simulink model "PowerAnalyserModel"  (R2026a)
settings: Solver=FixedStepAuto  StopTime=0.27  FixedStep=1e-5
libraries: eeRmsMeasurement x2, simulink x1
settings Model: Creator=Giulia  LastModifiedBy=Giulia

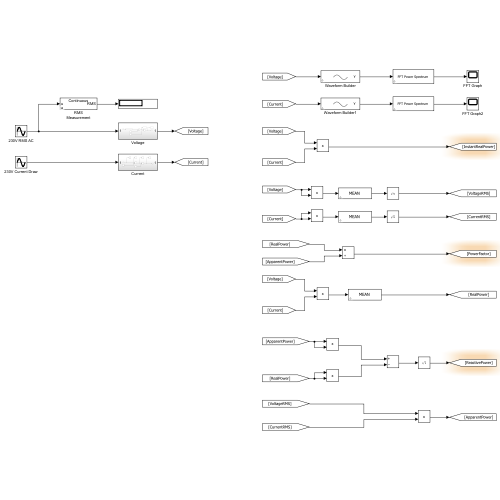
[thumbnail: Simulink's stored preview of the top-level diagram]
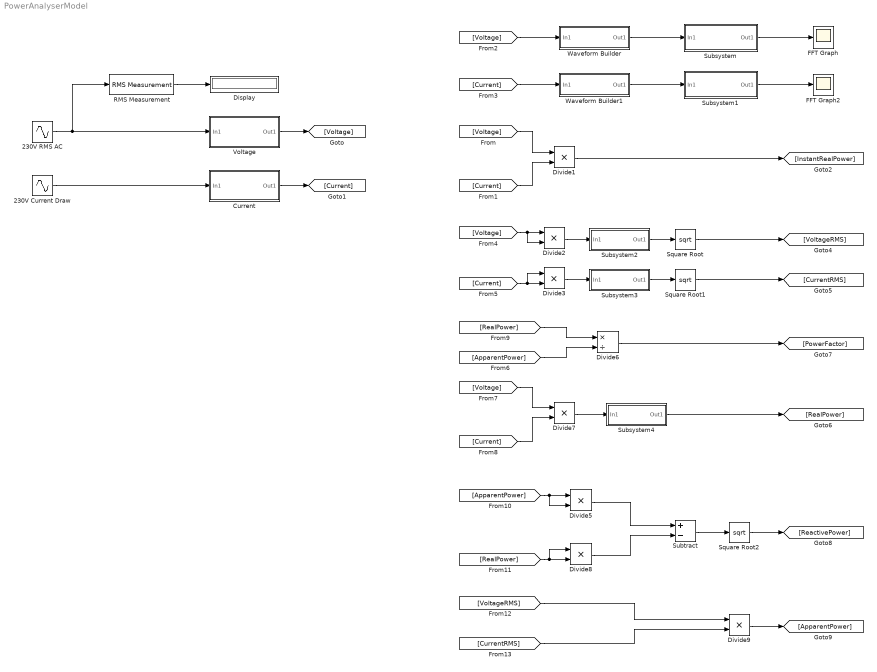
== system PowerAnalyserModel ==
  230V Current Draw : Sin  Amplitude=0.003  Frequency=50*pi*2  SampleTime=0
  230V RMS AC : Sin  Amplitude=325  Frequency=50*pi*2  SampleTime=0
  Current : Subsystem
  Display : Display
  Divide{1..3,5,7..9} (7 alike) : Product  Inputs=**
  Divide6 : Product  Inputs=*/
  FFT Graph : Scope
      settings: DataLoggingVariableName=ScopeData4
  FFT Graph2 : Scope
      settings: DataLoggingVariableName=ScopeData5
  RMS Measurement : eeRmsMeasurement/RMS Measurement  LabelModeActiveChoice=Total  F=50  SpecifyHarmonics=off  K=[0 1 2]  Ts=0
      settings: LibrarySourceBlock=|
      | ee_sl_lib/Measurements/RMS
      | Measurement
  Square Root : Sqrt
  Square Root1 : Sqrt
  Square Root2 : Sqrt
  Subsystem : Subsystem
  Subsystem1 : Subsystem
  Subsystem2 : Subsystem
  Subsystem3 : Subsystem
  Subsystem4 : Subsystem
  Subtract : Sum  Inputs=+-
  Voltage : Subsystem
  Waveform Builder : Subsystem
  Waveform Builder1 : Subsystem
  wires:
  230V RMS AC/1 -> Voltage/1(In1), RMS Measurement/1
  RMS Measurement/1 -> Display/1
  230V Current Draw/1 -> Current/1(In1)
  Voltage/1(Out1) -> [Voltage]
  Current/1(Out1) -> [Current]
  [Voltage] -> Divide1/1
  [Current] -> Divide1/2
  Divide1/1 -> [InstantRealPower]
  [Voltage] -> Waveform Builder/1(In1)
  Waveform Builder/1(Out1) -> Subsystem/1(In1)
  Subsystem/1(Out1) -> FFT Graph/1
  [Current] -> Waveform Builder1/1(In1)
  Waveform Builder1/1(Out1) -> Subsystem1/1(In1)
  Subsystem1/1(Out1) -> FFT Graph2/1
  [Voltage] -> Divide2/2, Divide2/1
  [Current] -> Divide3/1, Divide3/2
  Divide2/1 -> Subsystem2/1(In1)
  Divide3/1 -> Subsystem3/1(In1)
  Subsystem3/1(Out1) -> Square Root1/1
  Subsystem2/1(Out1) -> Square Root/1
  [ApparentPower] -> Divide6/2
  [Voltage] -> Divide7/1
  [Current] -> Divide7/2
  Divide7/1 -> Subsystem4/1(In1)
  Subsystem4/1(Out1) -> [RealPower]
  Square Root/1 -> [VoltageRMS]
  Square Root1/1 -> [CurrentRMS]
  [RealPower] -> Divide6/1
  Divide6/1 -> [PowerFactor]
  Square Root2/1 -> [ReactivePower]
  Subtract/1 -> Square Root2/1
  [ApparentPower] -> Divide5/2, Divide5/1
  Divide5/1 -> Subtract/1
  [RealPower] -> Divide8/1, Divide8/2
  Divide8/1 -> Subtract/2
  Divide9/1 -> [ApparentPower]
  [VoltageRMS] -> Divide9/1
  [CurrentRMS] -> Divide9/2

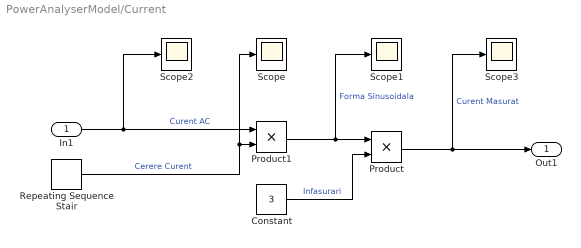
== system PowerAnalyserModel/Current ==
  In1 : Inport
  Constant : Constant  Value=3
  Product : Product
  Product1 : Product
  Repeating Sequence Stair : simulink/Sources/Repeating Sequence Stair  OutValues=[0 1 2 3 4 5 6 7 8 9 10 11 12 13].'  tsamp=0.02  OutMin=[]  OutMax=[]  OutDataTypeStr=double  OutputDataTypeScalingMode=double  OutDataType=fixdt(0,8)  ConRadixGroup=Best Precision: Vector-wise  OutScaling=2^-12
  Scope{,1..3} (4 alike) : Scope
      Scope settings: ActiveDisplayYMinimum=-1.6249999999999996  ActiveDisplayYMaximum=14.625
      Scope1 settings: ActiveDisplayYMinimum=-0.045375000000000006  ActiveDisplayYMaximum=0.048374999999999994
      Scope2 settings: ActiveDisplayYMinimum=-0.00375  ActiveDisplayYMaximum=0.00375  DataLoggingVariableName=ScopeData2
      Scope3 settings: ActiveDisplayYMinimum=-0.136125  ActiveDisplayYMaximum=0.145125  DataLoggingVariableName=ScopeData3
  Out1 : Outport
  wires:
  Constant/1 -> Product/2  "Infasurari"
  Product/1 -> Scope3/1, Out1/1  "Curent Masurat"
  Product1/1 -> Scope1/1, Product/1  "Forma Sinusoidala"
  In1/1 -> Product1/1, Scope2/1  "Curent AC"
  Repeating Sequence Stair/1 -> Scope/1, Product1/2  "Cerere Curent"

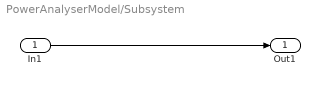
== system PowerAnalyserModel/Subsystem ==
  In1 : Inport
  Out1 : Outport
  wires:
  In1/1 -> Out1/1

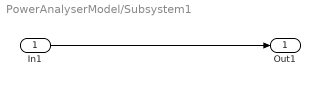
== system PowerAnalyserModel/Subsystem1 ==
  In1 : Inport
  Out1 : Outport
  wires:
  In1/1 -> Out1/1

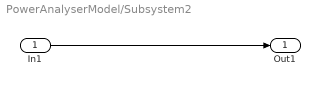
== system PowerAnalyserModel/Subsystem2 ==
  In1 : Inport
  Out1 : Outport
  wires:
  In1/1 -> Out1/1
  ? -> ?

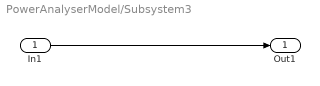
== system PowerAnalyserModel/Subsystem3 ==
  In1 : Inport
  Out1 : Outport
  wires:
  ? -> ?
  In1/1 -> Out1/1

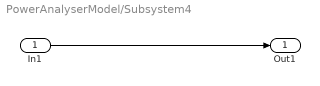
== system PowerAnalyserModel/Subsystem4 ==
  In1 : Inport
  Out1 : Outport
  wires:
  ? -> ?
  In1/1 -> Out1/1

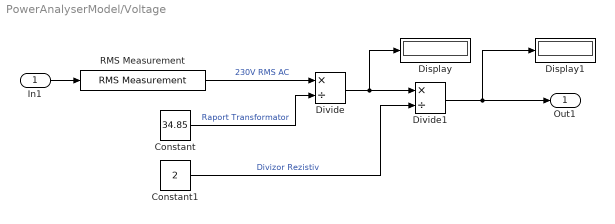
== system PowerAnalyserModel/Voltage ==
  In1 : Inport
  Constant : Constant  Value=34.85
  Constant1 : Constant  Value=2
  Display : Display
  Display1 : Display
  Divide : Product  Inputs=*/
  Divide1 : Product  Inputs=*/
  RMS Measurement : eeRmsMeasurement/RMS Measurement  LabelModeActiveChoice=Total  F=50  SpecifyHarmonics=off  K=[0 1 2]  Ts=0
      settings: LibrarySourceBlock=|
      | ee_sl_lib/Measurements/RMS
      | Measurement
  Out1 : Outport
  wires:
  In1/1 -> RMS Measurement/1
  Constant/1 -> Divide/2  "Raport Transformator"
  Divide/1 -> Display/1, Divide1/1
  Constant1/1 -> Divide1/2  "Divizor Rezistiv"
  Divide1/1 -> Display1/1, Out1/1
  RMS Measurement/1 -> Divide/1  "230V RMS AC"

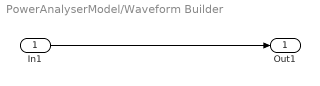
== system PowerAnalyserModel/Waveform Builder ==
  In1 : Inport
  Out1 : Outport
  wires:
  In1/1 -> Out1/1

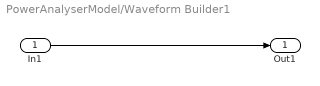
== system PowerAnalyserModel/Waveform Builder1 ==
  In1 : Inport
  Out1 : Outport
  wires:
  In1/1 -> Out1/1
